simulink model "Pacemaker"  (R2020a)
settings: Solver=FixedStepAuto  StartTime=0.0  StopTime=10.0  FixedStep=1e-3  RelTol=1e-3  EnableMultiTasking=on
undefined symbols (not defined in the file or in its folder): A3, A4, D0, D1, D10, D11, D12, D13, D2, D3, D5, D6, D8, D9, PTA0, PTA1, PTA2, PTB11, PTB9, PTC11, PTC16, PTC17, PTC2, PTC4, PTD0, PTD1, PTD2, PTD3
libraries: frdmk64flib x17, etargetslib x6
settings Model: ExtModeTrigDuration=5  Creator=USER  LastModifiedBy=USER
settings OptimizationCC: EnhancedBackFolding=on  PassReuseOutputArgsAs=Individual arguments  ZeroExternalMemoryAtStartup=off  ZeroInternalMemoryAtStartup=off  MaxStackSize=64  OptimizeBlockOrder=speed  DifferentSizesBufferReuse=on  OptimizationCustomize=off  EfficientTunableParamExpr=on
settings DebuggingCC: ParameterTunabilityLossMsg=error
settings HardwareCC: ProdBitPerPointer=32  ProdBitPerSizeT=32  ProdBitPerPtrDiffT=32  ProdLargestAtomicInteger=Long  ProdLargestAtomicFloat=Double  ProdWordSize=32  ProdHWDeviceType=ARM Compatible->ARM Cortex
settings SFSimCC: MATLABDynamicMemAlloc=off
settings RTWCC: SystemTargetFile=ert.tlc  HardwareBoard=NXP FRDM-K64F  TemplateMakefile=ert_default_tmf  Toolchain=GNU Tools for ARM Embedded Processors
settings CodeAppCC: ForceParamTrailComments=on  IgnoreCustomStorageClasses=off  OperatorAnnotations=on  SimulinkDataObjDesc=on  SFDataObjDesc=on  InsertBlockDesc=on

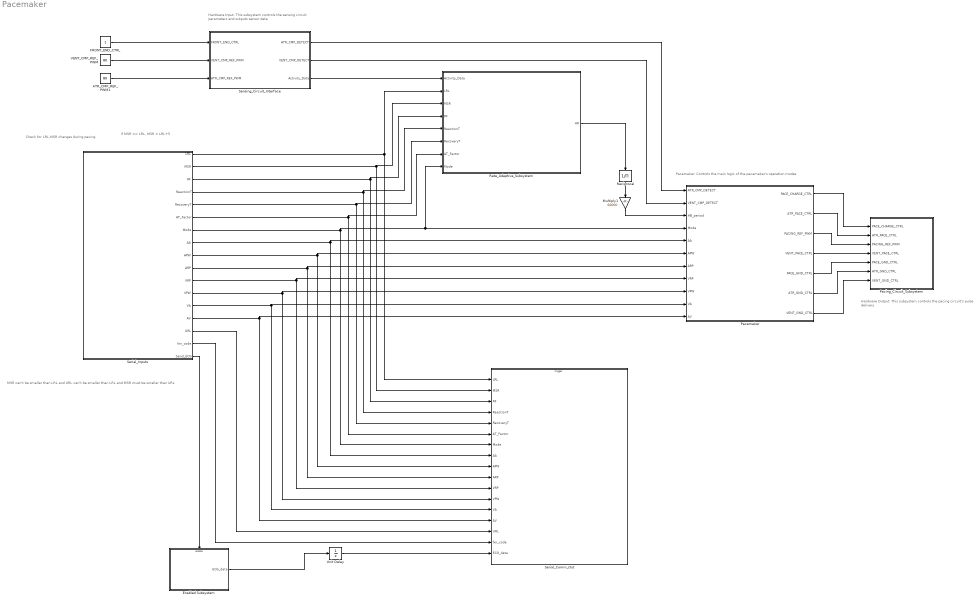
== system Pacemaker ==
  note: Check for LRL,MSR changes during pacing
  note: if MSR == LRL, MSR = LRL+5
  note: MSR can't be smaller than LRL and URL can't be smaller than LRL and MSR must be smaller than URL
  note: Pacemaker: Controls the main logic of the pacemaker's operation modes
  note: Hardware Input: This subsystem controls the sensing circuit parameters and outputs sensor data
  note: Hardware Output: This subsystem controls the pacing circuit's pulse delivery
  ATR_CMP_REF_PWM1 : Constant  Value=80  OutDataTypeStr=uint8
  Enabled Subsystem : Subsystem  TreatAsAtomicUnit=on
  FRONT_END_CTRL : Constant  OutDataTypeStr=boolean
  Multiply1 : Gain  Gain=60000  OutDataTypeStr=uint16  RndMeth=Round  SaturateOnIntegerOverflow=on
  Pacemaker : Stateflow chart  TreatAsAtomicUnit=on
      settings: PortSchema="{\"entries\":[{\"content\":{\"sides\":[{\"content\":{\"connectorIds\":[\"In2\",\"In3\",\"In10\",\"In1\",\"In6\",\"In8\",\"In4\",\"In5\",\"In9\",\"In7\",\"In11\"]},\"type\":\"ConnectorPlacement.EquallySpacedRectSide\",\"uuid\":\"be11ab42-f218-4533-b046-48d6c6672980\"},{\"content\":{\"connectorIds\":[\"Out1\",\"Out2\",\"Out3\",\"Out4\",\"Out5\",\"Out6\",\"Out7\"],\"side\":\"RIGHT\"},\"type\":\"ConnectorPlacement.EquallySpacedRectSide\",\"uuid\":\"3184d97a-d95e-4f92-be49-d512e0e8be59\"},{\"content\":{\"connectorIds\":[],\"side\":\"TOP\"},\"type\":\"ConnectorPlacement.EquallySpacedRectSide\",\"uuid\":\"82a667a0-8f6e-4fe8-9d7d-d285af85bcaa\"}]},\"type\":\"ConnectorPlacement.EquallySpacedConnector\",\"uuid\":\"8df3a08e-b350-4a50-854d-64d5d1a667ae\"}],\"packageUris\":[\"http://schema.mathworks.com/mf0/Connector/19700101\"],\"version\":\"1.0\"}"
  Pacing_Circuit_Subsystem : Subsystem
  Rate_Adaptive_Subsystem : Subsystem
  Reciprocal : Product  Inputs=/  OutDataTypeStr=double  RndMeth=Nearest
  Sensing_Circuit_Interface : Subsystem
  Serial_Comm_Out : Subsystem  TreatAsAtomicUnit=on
  Serial_Inputs : Subsystem
  Unit Delay : UnitDelay  SampleTime=-1  HasFrameUpgradeWarning=on
  VENT_CMP_REF_PWM : Constant  Value=80  OutDataTypeStr=uint8
  wires:
  Pacemaker/1(PACE_CHARGE_CTRL) -> Pacing_Circuit_Subsystem/1(PACE_CHARGE_CTRL)
  Pacemaker/2(ATR_PACE_CTRL) -> Pacing_Circuit_Subsystem/2(ATR_PACE_CTRL)
  Pacemaker/3(PACING_REF_PWM) -> Pacing_Circuit_Subsystem/3(PACING_REF_PWM)
  Pacemaker/4(VENT_PACE_CTRL) -> Pacing_Circuit_Subsystem/4(VENT_PACE_CTRL)
  Pacemaker/5(PACE_GND_CTRL) -> Pacing_Circuit_Subsystem/5(PACE_GND_CTRL)
  Pacemaker/6(ATR_GND_CTRL) -> Pacing_Circuit_Subsystem/6(ATR_GND_CTRL)
  Pacemaker/7(VENT_GND_CTRL) -> Pacing_Circuit_Subsystem/7(VENT_GND_CTRL)
  FRONT_END_CTRL/1 -> Sensing_Circuit_Interface/1(FRONT_END_CTRL)
  VENT_CMP_REF_PWM/1 -> Sensing_Circuit_Interface/2(VENT_CMP_REF_PWM)
  ATR_CMP_REF_PWM1/1 -> Sensing_Circuit_Interface/3(ATR_CMP_REF_PWM)
  Sensing_Circuit_Interface/1(ATR_CMP_DETECT) -> Pacemaker/2(ATR_CMP_DETECT)
  Sensing_Circuit_Interface/2(VENT_CMP_DETECT) -> Pacemaker/3(VENT_CMP_DETECT)
  Reciprocal/1 -> Multiply1/1
  Multiply1/1 -> Pacemaker/10(HB_period)
  Sensing_Circuit_Interface/3(Activity_Data) -> Rate_Adaptive_Subsystem/1(Activity_Data)
  Rate_Adaptive_Subsystem/1(HR) -> Reciprocal/1
  Serial_Inputs/7(Mode) -> Serial_Comm_Out/7(Mode), Rate_Adaptive_Subsystem/8(Mode), Pacemaker/1(Mode)
  Serial_Inputs/8(AA) -> Serial_Comm_Out/8(AA), Pacemaker/6(AA)
  Serial_Inputs/9(APW) -> Serial_Comm_Out/9(APW), Pacemaker/8(APW)
  Serial_Inputs/10(ARP) -> Serial_Comm_Out/10(ARP), Pacemaker/4(ARP)
  Serial_Inputs/11(VRP) -> Serial_Comm_Out/11(VRP), Pacemaker/5(VRP)
  Serial_Inputs/12(VPW) -> Serial_Comm_Out/12(VPW), Pacemaker/9(VPW)
  Serial_Inputs/13(VA) -> Serial_Comm_Out/13(VA), Pacemaker/7(VA)
  Serial_Inputs/14(AV) -> Serial_Comm_Out/14(AV), Pacemaker/11(AV)
  Serial_Inputs/16(fxn_code) -> Serial_Comm_Out/16(fxn_code)
  Serial_Inputs/1(LRL) -> Serial_Comm_Out/1(LRL), Rate_Adaptive_Subsystem/2(LRL)
  Serial_Inputs/15(URL) -> Serial_Comm_Out/15(URL)
  Serial_Inputs/2(MSR) -> Serial_Comm_Out/2(MSR), Rate_Adaptive_Subsystem/3(MSR)
  Serial_Inputs/3(RF) -> Serial_Comm_Out/3(RF), Rate_Adaptive_Subsystem/4(RF)
  Serial_Inputs/4(ReactionT) -> Serial_Comm_Out/4(ReactionT), Rate_Adaptive_Subsystem/5(ReactionT)
  Serial_Inputs/5(RecoveryT) -> Serial_Comm_Out/5(RecoveryT), Rate_Adaptive_Subsystem/6(RecoveryT)
  Serial_Inputs/6(AT_Factor) -> Serial_Comm_Out/6(AT_Factor), Rate_Adaptive_Subsystem/7(AT_Factor)
  Enabled Subsystem/1(ECG_data) -> Unit Delay/1
  Unit Delay/1 -> Serial_Comm_Out/17(ECG_data)
  Serial_Inputs/17(Send_ECG) -> Enabled Subsystem/Enable

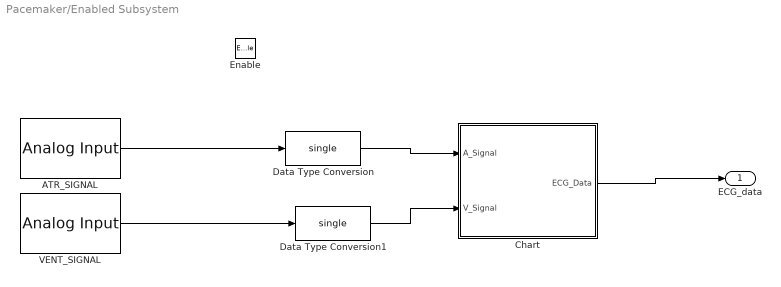
== system Pacemaker/Enabled Subsystem ==
  Enable : EnablePort
  ATR_SIGNAL : frdmk64flib/Analog Input  Whichpin=PTB11 (A3)  SampleTime=-1
  Chart : Stateflow chart  TreatAsAtomicUnit=on
  Data Type Conversion : DataTypeConversion  OutDataTypeStr=single
  Data Type Conversion1 : DataTypeConversion  OutDataTypeStr=single
  VENT_SIGNAL : frdmk64flib/Analog Input  Whichpin=PTC11 (A4)  SampleTime=-1
  ECG_data : Outport  OutDataTypeStr=single
  wires:
  Data Type Conversion/1 -> Chart/1(A_Signal)
  Data Type Conversion1/1 -> Chart/2(V_Signal)
  ATR_SIGNAL/1 -> Data Type Conversion/1
  VENT_SIGNAL/1 -> Data Type Conversion1/1
  Chart/1(ECG_Data) -> ECG_data/1

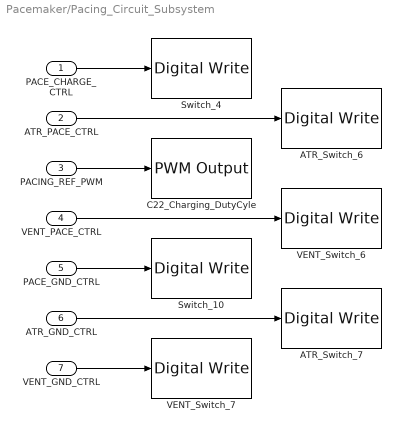
== system Pacemaker/Pacing_Circuit_Subsystem ==
  PACE_CHARGE_CTRL : Inport  OutDataTypeStr=boolean
  ATR_PACE_CTRL : Inport  Port=2  OutDataTypeStr=boolean
  PACING_REF_PWM : Inport  Port=3  OutDataTypeStr=uint8
  VENT_PACE_CTRL : Inport  Port=4  OutDataTypeStr=boolean
  PACE_GND_CTRL : Inport  Port=5  OutDataTypeStr=boolean
  ATR_GND_CTRL : Inport  Port=6  OutDataTypeStr=boolean
  VENT_GND_CTRL : Inport  Port=7  OutDataTypeStr=boolean
  ATR_Switch_6 : frdmk64flib/Digital Write  Whichpin=PTA0 (D8)
  ATR_Switch_7 : frdmk64flib/Digital Write  Whichpin=PTD2 (D11)
  C22_Charging_DutyCyle : frdmk64flib/PWM Output  Whichpin=PTA2 (D5)  InitialFrequency=2000  InitialDutyCycle=0
  Switch_10 : frdmk64flib/Digital Write  Whichpin=PTD0 (D10)
  Switch_4 : frdmk64flib/Digital Write  Whichpin=PTB9 (D2)
  VENT_Switch_6 : frdmk64flib/Digital Write  Whichpin=PTC4 (D9)
  VENT_Switch_7 : frdmk64flib/Digital Write  Whichpin=PTD3 (D12)
  wires:
  ATR_PACE_CTRL/1 -> ATR_Switch_6/1
  PACING_REF_PWM/1 -> C22_Charging_DutyCyle/1
  VENT_PACE_CTRL/1 -> VENT_Switch_6/1
  PACE_CHARGE_CTRL/1 -> Switch_4/1
  PACE_GND_CTRL/1 -> Switch_10/1
  VENT_GND_CTRL/1 -> VENT_Switch_7/1
  ATR_GND_CTRL/1 -> ATR_Switch_7/1

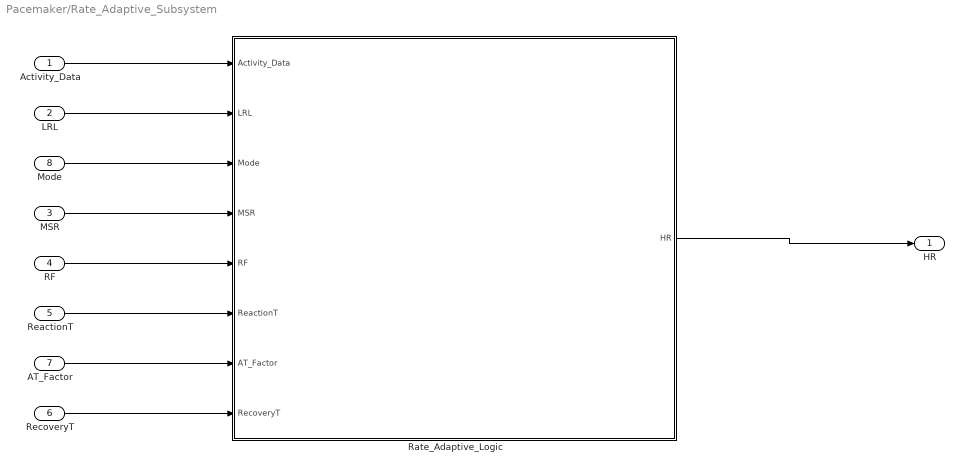
== system Pacemaker/Rate_Adaptive_Subsystem ==
  Activity_Data : Inport  OutDataTypeStr=double
  LRL : Inport  Port=2  OutDataTypeStr=uint8
  MSR : Inport  Port=3  OutDataTypeStr=uint8
  RF : Inport  Port=4  OutDataTypeStr=uint8
  ReactionT : Inport  Port=5  OutDataTypeStr=uint8
  RecoveryT : Inport  Port=6  OutDataTypeStr=uint8
  AT_Factor : Inport  Port=7  OutDataTypeStr=uint8
  Mode : Inport  Port=8  OutDataTypeStr=Enum: Modes
  Rate_Adaptive_Logic : Stateflow chart  TreatAsAtomicUnit=on
  HR : Outport  OutDataTypeStr=uint8
  wires:
  Activity_Data/1 -> Rate_Adaptive_Logic/1(Activity_Data)
  LRL/1 -> Rate_Adaptive_Logic/2(LRL)
  Mode/1 -> Rate_Adaptive_Logic/3(Mode)
  MSR/1 -> Rate_Adaptive_Logic/4(MSR)
  RF/1 -> Rate_Adaptive_Logic/5(RF)
  ReactionT/1 -> Rate_Adaptive_Logic/6(ReactionT)
  AT_Factor/1 -> Rate_Adaptive_Logic/7(AT_Factor)
  RecoveryT/1 -> Rate_Adaptive_Logic/8(RecoveryT)
  Rate_Adaptive_Logic/1(HR) -> HR/1

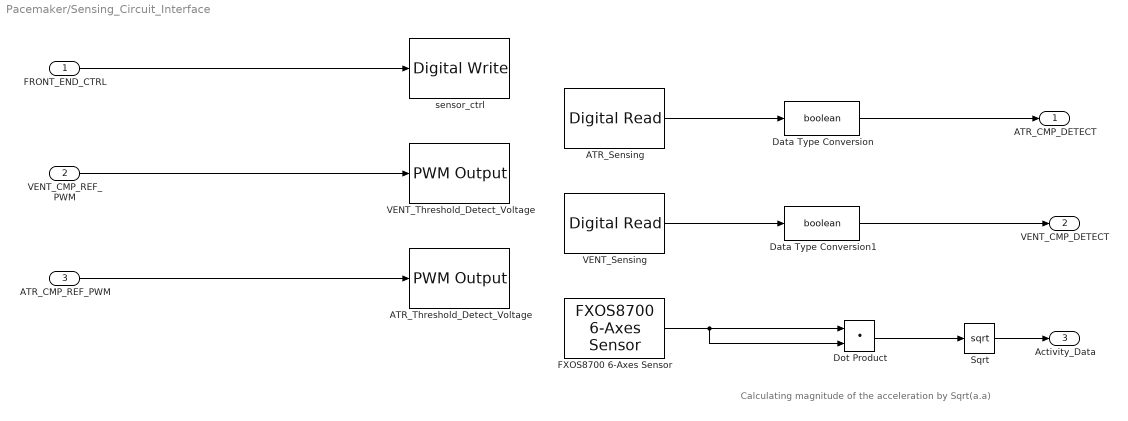
== system Pacemaker/Sensing_Circuit_Interface ==
  note: Calculating magnitude of the acceleration by Sqrt(a.a)
  FRONT_END_CTRL : Inport  OutDataTypeStr=boolean
  VENT_CMP_REF_PWM : Inport  Port=2  OutDataTypeStr=uint8
  ATR_CMP_REF_PWM : Inport  Port=3  OutDataTypeStr=uint8
  ATR_Sensing : frdmk64flib/Digital Read  Whichpin=PTC16 (D0)  SampleTime=-1
  ATR_Threshold_Detect_Voltage : frdmk64flib/PWM Output  Whichpin=PTC2 (D6)  InitialFrequency=2000  InitialDutyCycle=0
  Data Type Conversion : DataTypeConversion  OutDataTypeStr=boolean
  Data Type Conversion1 : DataTypeConversion  OutDataTypeStr=boolean
  Dot Product : DotProduct  OutDataTypeStr=double  InputSameDT=on
  FXOS8700 6-Axes Sensor : frdmk64flib/FXOS8700 6-Axes Sensor  Activesensor=Accelerometer only  ODR=800Hz  HybridODR=400Hz  Accelfullrange=-4g to +4g  SampleTime=-1
  Sqrt : Sqrt  OutDataTypeStr=double  SaturateOnIntegerOverflow=on
  VENT_Sensing : frdmk64flib/Digital Read  Whichpin=PTC17 (D1)  SampleTime=-1
  VENT_Threshold_Detect_Voltage : frdmk64flib/PWM Output  Whichpin=PTA1 (D3)  InitialFrequency=2000  InitialDutyCycle=0
  sensor_ctrl : frdmk64flib/Digital Write  Whichpin=PTD1 (D13)
  ATR_CMP_DETECT : Outport  OutDataTypeStr=boolean
  VENT_CMP_DETECT : Outport  Port=2  OutDataTypeStr=boolean
  Activity_Data : Outport  Port=3  OutDataTypeStr=double
  wires:
  VENT_Sensing/1 -> Data Type Conversion1/1
  ATR_Sensing/1 -> Data Type Conversion/1
  ATR_CMP_REF_PWM/1 -> ATR_Threshold_Detect_Voltage/1
  FRONT_END_CTRL/1 -> sensor_ctrl/1
  VENT_CMP_REF_PWM/1 -> VENT_Threshold_Detect_Voltage/1
  Data Type Conversion/1 -> ATR_CMP_DETECT/1
  Data Type Conversion1/1 -> VENT_CMP_DETECT/1
  Dot Product/1 -> Sqrt/1
  FXOS8700 6-Axes Sensor/1 -> Dot Product/2, Dot Product/1
  Sqrt/1 -> Activity_Data/1

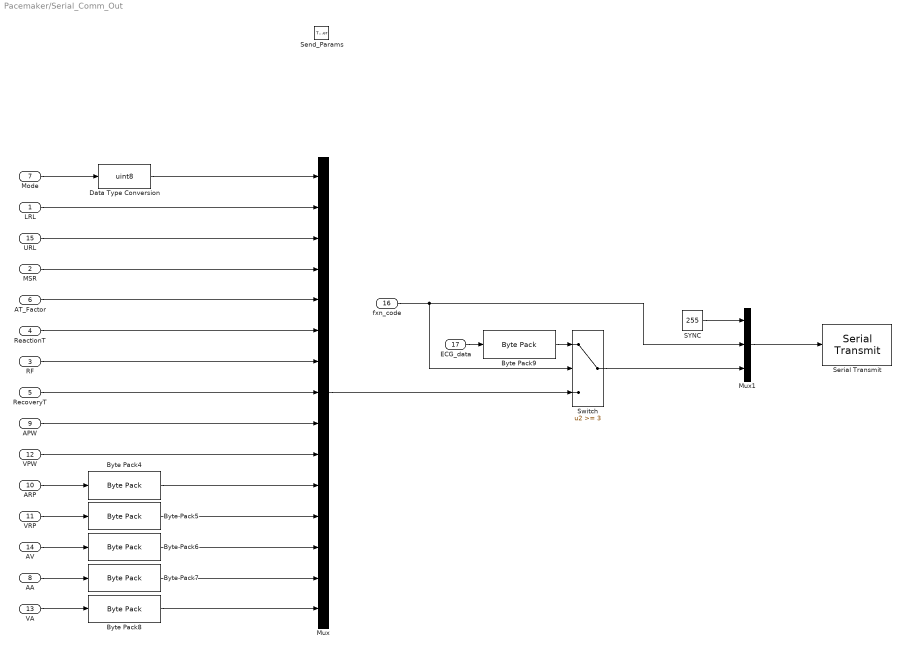
== system Pacemaker/Serial_Comm_Out ==
  LRL : Inport  OutDataTypeStr=uint8
  MSR : Inport  Port=2  OutDataTypeStr=uint8
  RF : Inport  Port=3  OutDataTypeStr=uint8
  ReactionT : Inport  Port=4  OutDataTypeStr=uint8
  RecoveryT : Inport  Port=5  OutDataTypeStr=uint8
  AT_Factor : Inport  Port=6  OutDataTypeStr=uint8
  Mode : Inport  Port=7  OutDataTypeStr=Enum: Modes
  AA : Inport  Port=8  OutDataTypeStr=single
  APW : Inport  Port=9  OutDataTypeStr=uint8
  ARP : Inport  Port=10  OutDataTypeStr=uint16
  VRP : Inport  Port=11  OutDataTypeStr=uint16
  VPW : Inport  Port=12  OutDataTypeStr=uint8
  VA : Inport  Port=13  OutDataTypeStr=single
  AV : Inport  Port=14  OutDataTypeStr=uint16
  URL : Inport  Port=15  OutDataTypeStr=uint8
  fxn_code : Inport  Port=16  OutDataTypeStr=uint8
  ECG_data : Inport  Port=17  OutDataTypeStr=single  PortDimensions=[1,6]
  Send_Params : TriggerPort  TriggerType=function-call  IsSimulinkFunction=on  FunctionName=Send_Params  VariantControl=Variant
  Byte Pack4 : etargetslib/Byte Pack  datatypes={'uint16'}  byteAlign=1
  Byte Pack5 : etargetslib/Byte Pack  datatypes={'uint16'}  byteAlign=1
  Byte Pack6 : etargetslib/Byte Pack  datatypes={'uint16'}  byteAlign=1
  Byte Pack7 : etargetslib/Byte Pack  datatypes={'single'}  byteAlign=1
  Byte Pack8 : etargetslib/Byte Pack  datatypes={'single'}  byteAlign=1
  Byte Pack9 : etargetslib/Byte Pack  datatypes={'single'}  byteAlign=1
  Data Type Conversion : DataTypeConversion  OutDataTypeStr=uint8
  Mux : Mux  Inputs=15
  Mux1 : Mux  Inputs=3
  SYNC : Constant  Value=255  OutDataTypeStr=uint8
  Serial Transmit : frdmk64flib/Serial Transmit  SCIModule=0  Baudrate=uint32(9600)  Parity=None  StopBits=1  HardwareFlowControl=None  ByteOrder=LittleEndian  BlockingMode=on  OutputStatus=off
  Switch : Switch  Threshold=3
  wires:
  Mode/1 -> Data Type Conversion/1
  URL/1 -> Mux/3
  MSR/1 -> Mux/4
  AT_Factor/1 -> Mux/5
  ReactionT/1 -> Mux/6
  RF/1 -> Mux/7
  RecoveryT/1 -> Mux/8
  APW/1 -> Mux/9
  VPW/1 -> Mux/10
  ARP/1 -> Byte Pack4/1
  VRP/1 -> Byte Pack5/1
  AV/1 -> Byte Pack6/1
  AA/1 -> Byte Pack7/1
  VA/1 -> Byte Pack8/1
  LRL/1 -> Mux/2
  Mux/1 -> Switch/3
  ECG_data/1 -> Byte Pack9/1
  fxn_code/1 -> Mux1/2, Switch/2
  Switch/1 -> Mux1/3
  SYNC/1 -> Mux1/1
  Mux1/1 -> Serial Transmit/1
  Byte Pack4/1 -> Mux/11
  Byte Pack5/1 -> Mux/12
  Byte Pack6/1 -> Mux/13
  Byte Pack7/1 -> Mux/14
  Byte Pack8/1 -> Mux/15
  Data Type Conversion/1 -> Mux/1
  Byte Pack9/1 -> Switch/1

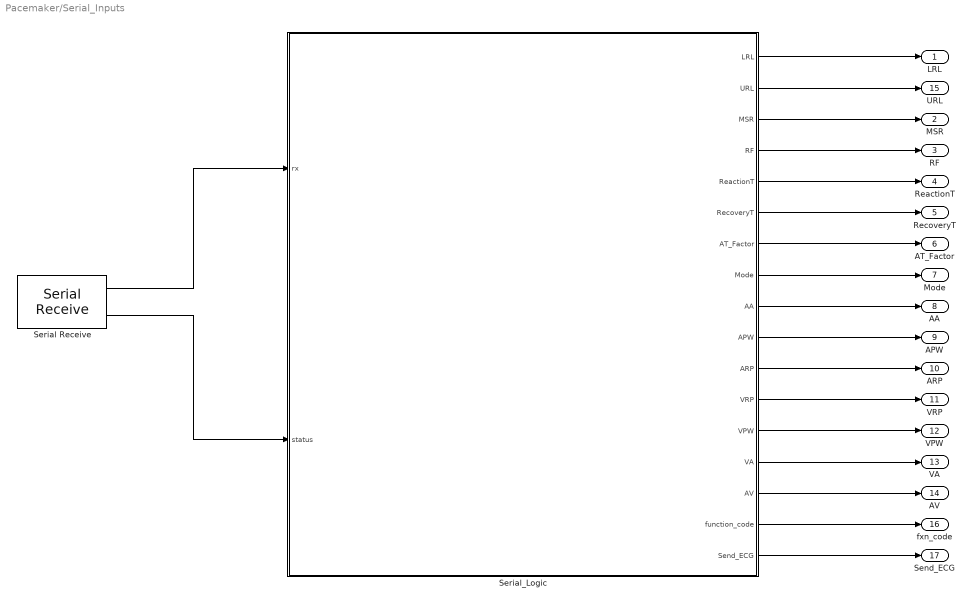
== system Pacemaker/Serial_Inputs ==
  Serial Receive : frdmk64flib/Serial Receive  SCIModule=0  Baudrate=uint32(9600)  Parity=None  StopBits=1  HardwareFlowControl=None  ByteOrder=LittleEndian  DataType=uint8  DataLength=26  BlockingMode=off  OutputStatus=on  SampleTime=0.1
  Serial_Logic : Stateflow chart  TreatAsAtomicUnit=on
      settings: PortSchema="{\"entries\":[{\"content\":{\"sides\":[{\"content\":{\"connectorIds\":[\"In1\",\"In2\"]},\"type\":\"ConnectorPlacement.EquallySpacedRectSide\",\"uuid\":\"65a5ff53-2abf-4eba-a904-12ba578282e4\"},{\"content\":{\"connectorIds\":[\"Out1\",\"Out16\",\"Out2\",\"Out3\",\"Out4\",\"Out5\",\"Out6\",\"Out7\",\"Out8\",\"Out9\",\"Out10\",\"Out11\",\"Out12\",\"Out13\",\"Out14\",\"Out15\",\"Out17\"],\"side\":\"RIGHT\"},\"type\":\"ConnectorPlacement.EquallySpacedRectSide\",\"uuid\":\"29128afb-6f79-493e-91f4-465b9e012737\"},{\"content\":{\"connectorIds\":[],\"side\":\"TOP\"},\"type\":\"ConnectorPlacement.EquallySpacedRectSide\",\"uuid\":\"8a5768ed-4891-46b2-bd94-4054f00e1a5a\"}]},\"type\":\"ConnectorPlacement.EquallySpacedConnector\",\"uuid\":\"2f56b7ef-6394-42fb-81a1-f2837d434a10\"}],\"packageUris\":[\"http://schema.mathworks.com/mf0/Connector/19700101\"],\"version\":\"1.0\"}"
  LRL : Outport  OutDataTypeStr=uint8
  MSR : Outport  Port=2  OutDataTypeStr=uint8
  RF : Outport  Port=3  OutDataTypeStr=uint8
  ReactionT : Outport  Port=4  OutDataTypeStr=uint8
  RecoveryT : Outport  Port=5  OutDataTypeStr=uint8
  AT_Factor : Outport  Port=6  OutDataTypeStr=uint8
  Mode : Outport  Port=7  OutDataTypeStr=Enum: Modes
  AA : Outport  Port=8  OutDataTypeStr=single
  APW : Outport  Port=9  OutDataTypeStr=uint8
  ARP : Outport  Port=10  OutDataTypeStr=uint16
  VRP : Outport  Port=11  OutDataTypeStr=uint16
  VPW : Outport  Port=12  OutDataTypeStr=uint8
  VA : Outport  Port=13  OutDataTypeStr=single
  AV : Outport  Port=14  OutDataTypeStr=uint16
  URL : Outport  Port=15
  fxn_code : Outport  Port=16  OutDataTypeStr=uint8
  Send_ECG : Outport  Port=17  OutDataTypeStr=boolean
  wires:
  Serial_Logic/1(LRL) -> LRL/1
  Serial_Logic/2(MSR) -> MSR/1
  Serial_Logic/3(RF) -> RF/1
  Serial_Logic/4(ReactionT) -> ReactionT/1
  Serial_Logic/5(RecoveryT) -> RecoveryT/1
  Serial_Logic/6(AT_Factor) -> AT_Factor/1
  Serial_Logic/7(Mode) -> Mode/1
  Serial_Logic/8(AA) -> AA/1
  Serial_Logic/9(APW) -> APW/1
  Serial_Logic/10(ARP) -> ARP/1
  Serial_Logic/11(VRP) -> VRP/1
  Serial_Logic/12(VPW) -> VPW/1
  Serial_Logic/13(VA) -> VA/1
  Serial_Logic/14(AV) -> AV/1
  Serial_Logic/15(function_code) -> fxn_code/1
  Serial Receive/1 -> Serial_Logic/1(rx)
  Serial Receive/2 -> Serial_Logic/2(status)
  Serial_Logic/16(URL) -> URL/1
  Serial_Logic/17(Send_ECG) -> Send_ECG/1

== stateflow chart Pacemaker/Pacemaker ==
  state AOO
    state Initial_ATR
      entry:
      % Charging C22 and Discharging C21
      ATR_PACE_CTRL = false;
      VENT_PACE_CTRL = false;
      PACING_REF_PWM = cast(AA*100/5,'uint8');
      PACE_CHARGE_CTRL = true;
      PACE_GND_CTRL = true;
      VENT_GND_CTRL = false;
      ATR_GND_CTRL = true;
      inPace = false;
    state Pace_ATR
      %This subchart is responsible for pacing the atrium
      state ATR_Pacing
        entry:
        %Discharging C22 through the heart
        PACE_CHARGE_CTRL = false;
        ATR_GND_CTRL = false;
        ATR_PACE_CTRL = true;
        inPace = true;
      state Charge_PaceC_Discharge_BlockingC
        entry:
        %Charging C22 and Discharging C21
        %Setting PACING_REF PWM is not needed since
        %it didn't change from the initial state
        ATR_PACE_CTRL = false;
        VENT_PACE_CTRL = false;
        PACE_CHARGE_CTRL = true;
        PACE_GND_CTRL = true;
        VENT_GND_CTRL = false;
        ATR_GND_CTRL = true;
        inPace = false;
      (default) -> AOO.Pace_ATR.ATR_Pacing
      AOO.Pace_ATR.ATR_Pacing -> AOO.Pace_ATR.Charge_PaceC_Discharge_BlockingC : after(APW,msec)
    note: Initial delay to charge C22
    (default) -> AOO.Initial_ATR
    AOO.Initial_ATR -> AOO.Pace_ATR : after(HB_period,msec)
    AOO.Pace_ATR -> AOO.Pace_ATR : after(HB_period,msec)
  note: Pace_ATR and Pace_VENT are subcharts which are responsible for delivering a single artificial pulse to the atrium and ventricle respectively
  state VOO
    state Initial_VENT
      entry:
      %Charging C22 and Discharging C21
      ATR_PACE_CTRL = false;
      VENT_PACE_CTRL = false;
      PACING_REF_PWM = cast(VA*100/5,'uint8');
      PACE_CHARGE_CTRL = true;
      PACE_GND_CTRL = true;
      ATR_GND_CTRL = false;
      VENT_GND_CTRL = true;
      inPace = false;
    note: Initial delay to charge C22
    state Pace_VENT
      %This subchart is for pacing the ventricle
      state VENT_Pacing
        entry:
        %Discharging C22 through the heart
        PACE_CHARGE_CTRL=false;
        VENT_GND_CTRL=false;
        VENT_PACE_CTRL=true;
        inPace = true;
      state Charge_PaceC_Discharge_Discharge_BlockingC
        entry:
        %Charging C22 and Discharging C21
        %Setting PACING_REF PWM is not needed since
        %it didn't change from the initial state
        ATR_PACE_CTRL = false;
        VENT_PACE_CTRL = false;
        PACE_CHARGE_CTRL = true;
        PACE_GND_CTRL = true;
        ATR_GND_CTRL=false;
        VENT_GND_CTRL = true;
        inPace = false;
      (default) -> VOO.Pace_VENT.VENT_Pacing
      VOO.Pace_VENT.VENT_Pacing -> VOO.Pace_VENT.Charge_PaceC_Discharge_Discharge_BlockingC : after(VPW,msec)
    (default) -> VOO.Initial_VENT
    VOO.Initial_VENT -> VOO.Pace_VENT : after(HB_period,msec)
    VOO.Pace_VENT -> VOO.Pace_VENT : after(HB_period,msec)
  state No_Pace
    %Setting default values of parameters
    PACE_CHARGE_CTRL = false;
    ATR_PACE_CTRL = false;
    PACING_REF_PWM = 0;
    VENT_PACE_CTRL = false;
    PACE_GND_CTRL = true;
    ATR_GND_CTRL = true;
    VENT_GND_CTRL = true;
    inPace = false;
    %HB_period = 1000/(cast(LRL,'uint16')/60);
  note: The inPace variable is used to avoid switching modes while delivering a pace (explained in pacemaker documentation)
  state VVI
    state Initial_VENT
      entry:
      %Charging C22 and Discharging C21
      ATR_PACE_CTRL = false;
      VENT_PACE_CTRL = false;
      PACING_REF_PWM = cast(VA*100/5,'uint8');
      PACE_CHARGE_CTRL = true;
      PACE_GND_CTRL = true;
      ATR_GND_CTRL = false;
      VENT_GND_CTRL = true;
      inPace = false;
    state Sense
      %{
      In this state we wait to sense a natural pulse from
      the heart. If the heart sends a pulse within
      (heart beat period - refractory period), we
      send inhibit the pace and go to the wait state.
      Else, we send an artificial pulse to the heart
      %}
    state wait_NP
      %{
      We enter this state if we
      detect a natural pulse from
      the heart and ignore all
      incoming heart signals for the
      duration of the refractory period
      %}
    state Pace_VENT
      %This subchart is for pacing the ventricle
      state VENT_Pacing
        entry:
        %Discharging C22 through the heart
        PACE_CHARGE_CTRL=false;
        VENT_GND_CTRL=false;
        VENT_PACE_CTRL=true;
        inPace = true;
      state Charge_PaceC_Discharge_Discharge_BlockingC
        entry:
        %Charging C22 and Discharging C21
        %Setting PACING_REF PWM is not needed since
        %it didn't change from the initial state
        ATR_PACE_CTRL = false;
        VENT_PACE_CTRL = false;
        PACE_CHARGE_CTRL = true;
        PACE_GND_CTRL = true;
        ATR_GND_CTRL=false;
        VENT_GND_CTRL = true;
        inPace = false;
      (default) -> VVI.Pace_VENT.VENT_Pacing
      VVI.Pace_VENT.VENT_Pacing -> VVI.Pace_VENT.Charge_PaceC_Discharge_Discharge_BlockingC : after(VPW,msec)
    VVI.Sense -> VVI.wait_NP [order 1] : [VENT_CMP_DETECT == true]
    (default) -> VVI.Initial_VENT
    VVI.wait_NP -> VVI.Sense : after(VRP,msec)
    VVI.Initial_VENT -> VVI.Sense
    VVI.Sense -> VVI.Pace_VENT [order 2] : after(HB_period-VRP,msec)
    VVI.Pace_VENT -> VVI.Sense : after(VRP,msec)
  state AAI
    state Initial_ATR
      entry:
      % Charging C22 and Discharging C21
      ATR_PACE_CTRL = false;
      VENT_PACE_CTRL = false;
      PACING_REF_PWM = cast(AA*100/5,'uint8');
      PACE_CHARGE_CTRL = true;
      PACE_GND_CTRL = true;
      VENT_GND_CTRL = false;
      ATR_GND_CTRL = true;
      inPace = false;
    state Sense
      %{
      In this state we wait to sense a natural pulse from
      the heart. If the heart sends a pulse within
      (heart beat period - refractory period), we
      send inhibit the pace and go to the wait state.
      Else, we send an artificial pulse to the heart
      %}
    state wait_NP
      %{
      We enter this state if we
      detect a natural pulse from
      the heart and ignore all
      incoming heart signals for the
      duration of the refractory period
      %}
    state Pace_ATR
      %This subchart is responsible for pacing the atrium
      state ATR_Pacing
        entry:
        %Discharging C22 through the heart
        PACE_CHARGE_CTRL = false;
        ATR_GND_CTRL = false;
        ATR_PACE_CTRL = true;
        inPace = true;
      state Charge_PaceC_Discharge_BlockingC
        entry:
        %Charging C22 and Discharging C21
        %Setting PACING_REF PWM is not needed since
        %it didn't change from the initial state
        ATR_PACE_CTRL = false;
        VENT_PACE_CTRL = false;
        PACE_CHARGE_CTRL = true;
        PACE_GND_CTRL = true;
        VENT_GND_CTRL = false;
        ATR_GND_CTRL = true;
        inPace = false;
      (default) -> AAI.Pace_ATR.ATR_Pacing
      AAI.Pace_ATR.ATR_Pacing -> AAI.Pace_ATR.Charge_PaceC_Discharge_BlockingC : after(APW,msec)
    (default) -> AAI.Initial_ATR
    AAI.Sense -> AAI.wait_NP [order 2] : [ATR_CMP_DETECT == true]
    AAI.Initial_ATR -> AAI.Sense
    AAI.wait_NP -> AAI.Sense : after(ARP,msec)
    AAI.Sense -> AAI.Pace_ATR [order 1] : after(HB_period - ARP,msec)
    AAI.Pace_ATR -> AAI.Sense : after(ARP,msec)
  state DOO
    state Initial_ATR
      entry:
      % Charging C22 and Discharging C21
      ATR_PACE_CTRL = false;
      VENT_PACE_CTRL = false;
      PACING_REF_PWM = cast(AA*100/5,'uint8');
      PACE_CHARGE_CTRL = true;
      PACE_GND_CTRL = true;
      VENT_GND_CTRL = false;
      ATR_GND_CTRL = true;
      inPace = false;
    state Pace_ATR
      %This subchart is responsible for pacing the atrium
      state ATR_Pacing
        entry:
        %Discharging C22 through the heart
        PACE_CHARGE_CTRL = false;
        ATR_GND_CTRL = false;
        ATR_PACE_CTRL = true;
        inPace = true;
      state Initial_VENT
        entry:
        %Charging C22 and Discharging C21
        ATR_PACE_CTRL = false;
        VENT_PACE_CTRL = false;
        PACING_REF_PWM = cast(VA*100/5,'uint8');
        PACE_CHARGE_CTRL = true;
        PACE_GND_CTRL = true;
        ATR_GND_CTRL = false;
        VENT_GND_CTRL = true;
        inPace = false;
      (default) -> DOO.Pace_ATR.ATR_Pacing
      DOO.Pace_ATR.ATR_Pacing -> DOO.Pace_ATR.Initial_VENT : after(APW,msec)
    state Pace_VENT
      %This subchart is for pacing the ventricle
      state VENT_Pacing
        entry:
        %Discharging C22 through the heart
        PACE_CHARGE_CTRL=false;
        VENT_GND_CTRL=false;
        VENT_PACE_CTRL=true;
        inPace = true;
      state Charge_PaceC_Discharge_BlockingC
        entry:
        %Charging C22 and Discharging C21
        %Setting PACING_REF PWM is not needed since
        %it didn't change from the initial state
        ATR_PACE_CTRL = false;
        VENT_PACE_CTRL = false;
        PACE_CHARGE_CTRL = true;
        PACE_GND_CTRL = true;
        VENT_GND_CTRL = false;
        ATR_GND_CTRL = true;
        inPace = false;
      (default) -> DOO.Pace_VENT.VENT_Pacing
      DOO.Pace_VENT.VENT_Pacing -> DOO.Pace_VENT.Charge_PaceC_Discharge_BlockingC : after(VPW,msec)
    (default) -> DOO.Initial_ATR
    DOO.Initial_ATR -> DOO.Pace_ATR : after(HB_period-AV,msec)
    DOO.Pace_VENT -> DOO.Pace_ATR : after(HB_period-AV,msec)
    DOO.Pace_ATR -> DOO.Pace_VENT : after(AV,msec)
  (default) -> No_Pace
  (junction 22) -> AOO [order 3] : [Mode == Modes.AOO]
  AOO -> (junction 22) : [Mode ~=Modes.AOO && inPace == false]
  VOO -> (junction 22) : [Mode ~= Modes.VOO  && inPace == false]
  No_Pace -> (junction 22) : [Mode ~= Modes.NO_PACE]
  (junction 22) -> VOO [order 4] : [Mode == Modes.VOO]
  (junction 22) -> No_Pace [order 1] : [Mode == Modes.NO_PACE]
  (junction 22) -> VVI [order 5] : [Mode == Modes.VVI]
  (junction 22) -> AAI [order 6] : [Mode == Modes.AAI]
  AAI -> (junction 22) : [Mode ~= Modes.AAI  && inPace == false]
  (junction 22) -> DOO [order 2] : [Mode==Modes.DOO]
  DOO -> (junction 22) : [Mode ~= Modes.DOO && inPace == false]
  VVI -> (junction 22) : [Mode ~= Modes.VVI  && inPace == false]
  data: Mode input Enum: Modes; ATR_CMP_DETECT input boolean; VENT_CMP_DETECT input boolean; ARP input uint16; VRP input uint16; AA input single; VA input single; APW input uint8; VPW input uint8; PACE_CHARGE_CTRL output boolean; ATR_PACE_CTRL output boolean; PACING_REF_PWM output uint8; VENT_PACE_CTRL output boolean; PACE_GND_CTRL output boolean; ATR_GND_CTRL output boolean; VENT_GND_CTRL output boolean; HB_period input uint16; AV input uint16; inPace local boolean

== stateflow chart Pacemaker/Serial_Inputs/Serial_Logic ==
  settings: executeAtInitialization=1
  state Serial_Receive
    state Echo_params
      en:
      Send_Params();
    state Send_ECG
      entry:
      Send_ECG = true;
    state Initialize
      en:
      LRL = 60;
      URL = 120;
      MSR = 120;
      RF = 8;
      ReactionT = 30;
      RecoveryT = 2;
      AT_Factor = 4;
      Mode = Modes.NO_PACE;
      AA = 3.5;
      VA = 3.5;
      APW = 2;
      VPW = 2;
      ARP = 250;
      VRP = 320;
      AV = 150;
    state Standby
      %Waiting for Com
    state Check_function_code
      en:
      function_code = rx(2);
      rx_to_save = rx;
    state Stop__ECG
      entry:
      Send_ECG = false;
    state Write_params
      en:
      %[Sync,fxn_code,MODE, LRL, URL, MSR, AT, ReactionT, RF, RecoveryT, APW, VPW, ARP, VRP, AV, AA, VA]
      Mode = Modes(rx_to_save(3));
      %Check that LRL<MSR <= URL, otherwise, hold previous values
      if (rx_to_save(4) < rx_to_save(6) && rx_to_save(6) <= rx_to_save(5))
      LRL = rx_to_save(4);
      URL = rx_to_save(5);
      MSR = rx_to_save(6);
      end
      AT_Factor = rx_to_save(7);
      ReactionT = rx_to_save(8);
      RF = rx_to_save(9);
      RecoveryT = rx_to_save(10);
      APW = rx_to_save(11);
      VPW = rx_to_save(12);
      ARP = typecast(rx_to_save(13:14),'uint16');
      VRP = typecast(rx_to_save(15:16),'uint16');
      AV = typecast(rx_to_save(17:18),'uint16');
      AA = typecast(rx_to_save(19:22),'single');
      VA = typecast(rx_to_save(23:26),'single');
    Send_ECG -> Standby
    Echo_params -> Standby
    (default) -> Initialize
    Check_function_code -> Send_ECG [order 3] : [function_code == 3]
    Check_function_code -> Echo_params [order 1] : [function_code == 1]
    (junction 96) -> Standby [order 2]
    Initialize -> Standby
    Standby -> (junction 96) : [status == 0]
    (junction 96) -> Check_function_code [order 1] : [rx(1) == 255]
    Check_function_code -> Stop__ECG [order 4] : [function_code == 4]
    Write_params -> Standby
    Stop__ECG -> Standby
    Check_function_code -> Standby [order 5]
    Check_function_code -> Write_params [order 2] : [function_code == 2]
  data: LRL output uint8; MSR output uint8; RF output uint8; ReactionT output uint8; RecoveryT output uint8; AT_Factor output uint8; Mode output Enum: Modes; AA output single; APW output uint8; ARP output uint16; VRP output uint16; VPW output uint8; VA output single; AV output uint16; rx input uint8; status input uint8; rx_to_save local uint8 size=[26,1]; function_code output uint8; URL output uint8; Send_ECG output boolean

== stateflow chart Pacemaker/Rate_Adaptive_Subsystem/Rate_Adaptive_Logic ==
  state Nonadaptive
    entry:
    HR = LRL;
  state Update_Target_Chart [commented out]
    state Not_Active_Enough [commented out]
      entry:
      Target_HR = LRL;
    state Find_Target [commented out]
      entry:
      c = 1;
      Target_HR = LRL + ...
      cast(RF*c*(activity_avg - Activity_Threshold),'uint8');
      if (Target_HR < LRL) Target_HR = LRL;
      elseif (Target_HR > MSR) Target_HR = MSR;
      end
    (default) -> Not_Active_Enough [commented out]
    Not_Active_Enough -> Find_Target [commented out] : [activity_avg > Activity_Threshold]
    Find_Target -> Not_Active_Enough [commented out] : [activity_avg <= Activity_Threshold]
  state Rate_Adaptive
    state Finding_Activity_AVG [parallel]
      settings: executionOrder=1
      state Initialize
        entry:
        sampling_time = 20;
        activity_avg = 1;
        sum_activity = 0;
        counter = 0;
        sampling_interval = 100;
        max_samples = sampling_time*1000/sampling_interval;
        c = 5.3;
        Activity_Threshold = 1+0.05*cast(AT_Factor,'double');
      state Sample
        entry:
        sum_activity = sum_activity + Activity_Data;
        counter = counter + 1;
      state Finding_AVG
        entry:
        activity_avg = sum_activity/cast(counter,'double');
        sum_activity = 0;
        counter = 0;
        Update_Target();
        target_changed = true;
      (default) -> Rate_Adaptive.Finding_Activity_AVG.Initialize
      Sample -> Sample [order 1] : after(sampling_interval,msec)
      Rate_Adaptive.Finding_Activity_AVG.Initialize -> Sample
      Finding_AVG -> Sample
      Sample -> Finding_AVG [order 2] : [counter == max_samples]
    state Update_Target [function]
      (default) -> (junction 68)
      (junction 68) -> (junction 72) [order 1] : [activity_avg <= Activity_Threshold]{Target_HR = LRL;}
      (junction 68) -> (junction 74) [order 2] : {
          | Target_HR = LRL + ...
          | cast(RF*c*(activity_avg - Activity_Threshold),'uint8');
          | }
      (junction 74) -> (junction 78) : [Target_HR > MSR]{Target_HR = MSR;}
      (junction 74) -> (junction 76) [commented out] : [Target_HR<LRL]{Target_HR = LRL;}
    state Update_HR [parallel]
      settings: executionOrder=2
      state Increment_Initialization
        entry:
        time_to_reach_target = cast(ReactionT,'double')/cast((MSR-LRL),'double') * cast((Target_HR-prev_HR),'double');
        n = cast(time_to_reach_target/time_step_reaction,'uint8');
        increment = (Target_HR - prev_HR)/n;
      state Check
        en:
        target_changed = false;
        prev_HR = HR;
      state Initialize
        entry:
        time_step_reaction = 0.5;
        time_step_recovery = 5;
      state Increment_HR
        en:
        HR = HR+increment;
      state Decrement
        en:
        time_to_reach_target = cast(RecoveryT,'double')*60/cast((MSR-LRL),'double') * cast((prev_HR-Target_HR),'double');
        n = cast(time_to_reach_target/time_step_recovery,'uint8');
        decrement = (prev_HR-Target_HR)/n;
      state Decrement_HR
        en:
        HR = HR-decrement;
      (default) -> Rate_Adaptive.Update_HR.Initialize
      Check -> Increment_Initialization [order 1] : [prev_HR < Target_HR]
      Rate_Adaptive.Update_HR.Initialize -> Check
      Increment_HR -> Check [order 2] : [target_changed == true || HR >= Target_HR]
      Increment_Initialization -> Increment_HR
      Check -> Decrement [order 2] : [prev_HR > Target_HR]
      Decrement_HR -> Check [order 1] : [target_changed == true || HR <= Target_HR]
      Increment_HR -> Increment_HR [order 1] : after(time_step_reaction,sec)
      Decrement -> Decrement_HR
      Decrement_HR -> Decrement_HR [order 2] : after(time_step_recovery,sec)
  state Rate_Adaptive1 [commented out]
    %{
    Obtain Target_HR
    {
    (Repeat every sampling_time seconds)
    Sample Activity Data for sampling_time seconds #sampling_time = 10-30 s
    and take an average to determine activity_avg
    if (activity_avg <= threshold) Target_HR = LRL;
    else
    slope = RF*c;
    Target_HR = LRL + slope*(activity_avg - threshold);
    if (Target_HR > MSR) Ta rget_HR = MSR;
    previous = HR;
    }
    Increment Actual HR
    {
    if (previous < Target_HR)
    {
    time_to_reach_Target = ReactionT/(MSR-LRL) * (target-previous);
    n = time_to_reach_Target/time_step; #time_step_reaction = 500 ms;
    for (i = 0; i<sampling_time/(time_step_reaction); i = i + 1)
    {
    HR = HR + (target-previous)/n;
    delay(time_step_reaction);
    }
    }
    if (previous > Target_HR)
    {
    time_to_reach_Target = RecoveryT/(MSR-LRL) * (previous - target);
    n = time_to_reach_Target/time_step; #time_step_recovery = 5 s;
    for (i = 0; i<sampling_time/(time_step); i = i + 1)
    {
    HR = HR + (target-previous)/n;
    delay(time_step_recovery);
    }
    }
    }
    %}
  (default) -> Nonadaptive
  Rate_Adaptive -> Nonadaptive : [Mode == Modes.AOO || ...
      | Mode == Modes.VOO || ...
      | Mode == Modes.AAI || ...
      |  Mode == Modes.VVI || ...
      |  Mode == Modes. DOO]
  Nonadaptive -> Rate_Adaptive : [Mode == Modes.AOOR || ...
      | Mode == Modes.VOOR || ...
      | Mode == Modes.AAIR || ...
      |  Mode == Modes.VVIR || ...
      |  Mode == Modes. DOOR]
  data: c local double; sum_activity local double; counter local uint16; sampling_interval local uint16; max_samples local uint16; sampling_time local uint16; decrement local uint8; increment local uint8; n local uint8; time_step_reaction local double; time_step_recovery local double; time_to_reach_target local double; Target_HR local uint8; activity_avg local double; c local double; prev_HR local uint8; target_changed local boolean; Activity_Data input double; LRL input uint8; Mode input Enum: Modes; MSR input uint8; RF input uint8; ReactionT input uint8; AT_Factor input uint8; RecoveryT input uint8; HR output uint8; Activity_Threshold local double

== stateflow chart Pacemaker/Enabled Subsystem/Chart ==
  settings: updateMethod=DISCRETE  sampleTime=0.1  initializeOutput=1
  state Sampling
    en:
    ECG_Data(counter) = A_Signal;
    ECG_Data(counter+1) = V_Signal;
    counter = counter + 2;
  state Initialize
    en:
    ECG_Data = zeros(1,6);
    counter = 1;
    sampling_interval = 2;
  (default) -> Initialize
  Sampling -> Sampling [order 2] : after(sampling_interval,msec)
  Initialize -> Sampling
  Sampling -> Initialize [order 1] : [counter == 7]{Send_Params();}
  data: A_Signal input single; V_Signal input single; ECG_Data output single size=[1,6]; sampling_interval local uint16; counter local uint8
